simulink model "AB2L2v2015a"  (R2015a)
settings: Solver=ode45  SolverMode=SingleTasking  StartTime=0.0  StopTime=40.0  RelTol=1e-3
settings Model: CovMetricSettings=dwe  CovHtmlReporting=off  covSaveCumulativeToWorkspaceVar=off  CovSaveSingleToWorkspaceVar=off  CovExternalEMLEnable=on  Creator=root  LastModifiedBy=root
settings DataIOCC: LimitDataPoints=off  SaveFormat=Dataset
settings DebuggingCC: SFUnexpectedBacktrackingDiag=error  SFNoUnconditionalDefaultTransitionDiag=error
settings HardwareCC: ProdBitPerPointer=64  ProdLargestAtomicFloat=Float  ProdIntDivRoundTo=Zero  ProdEndianess=LittleEndian  ProdHWDeviceType=Specified
settings ModelReferenceCC: PropagateSignalLabelsOutOfModel=on
settings SFSimCC: SimUseLocalCustomCode=on
settings RTWCC: RTWUseLocalCustomCode=on
settings GRTTargetCC: TargetLangStandard=C99 (ISO)  GeneratePreprocessorConditionals=Use local settings

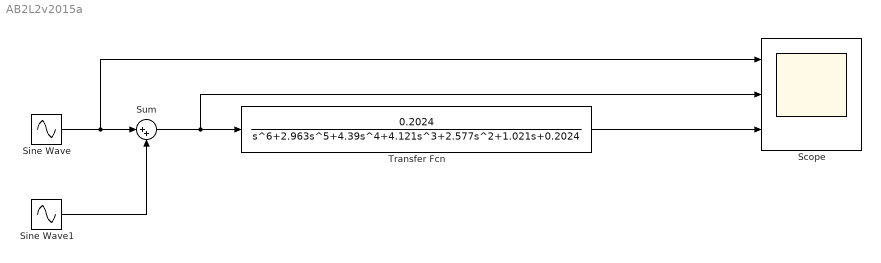
== system AB2L2v2015a ==
  Scope : Scope  NumInputPorts=3
      settings: TimeRange=auto  ShowLegends=on  MaxDataPoints=5000  SaveToWorkspace=off  SaveName=ScopeData  YMin=-1.35067~-5~-5  YMax=1.36371~5~5  SampleTime=-1
  Sine Wave : Sin  Frequency=.225*pi  SampleTime=0
  Sine Wave1 : Sin  Amplitude=.1  Frequency=10*pi  SampleTime=0
  Sum : Sum  Inputs=|++
  Transfer Fcn : TransferFcn  Numerator=0.2024  Denominator=[1 2.963 4.39 4.121 2.577 1.021 0.2024]
  wires:
  Sine Wave/1 -> Scope/1, Sum/1
  Sine Wave1/1 -> Sum/2
  Sum/1 -> Scope/2, Transfer Fcn/1
  Transfer Fcn/1 -> Scope/3
